simulink model "task8.1"  (R2023b)
settings: Solver=VariableStepAuto  StartTime=0.0  StopTime=2000  RelTol=1e-3
undefined symbols (not defined in the file or in its folder): SS_lat_lo8
libraries: slpidlib x5
settings Model: Creator=antonhendrickx  LastModifiedBy=antonhendrickx

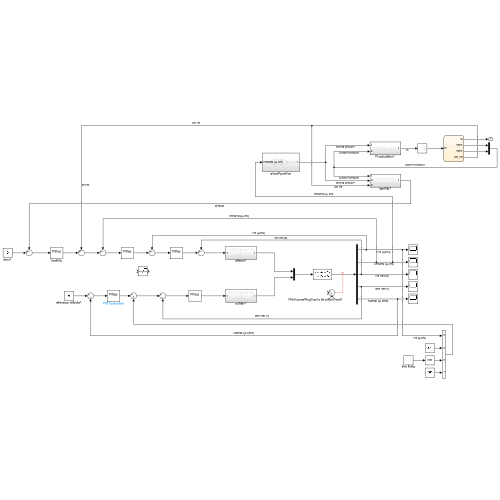
[thumbnail: Simulink's stored preview of the top-level diagram]
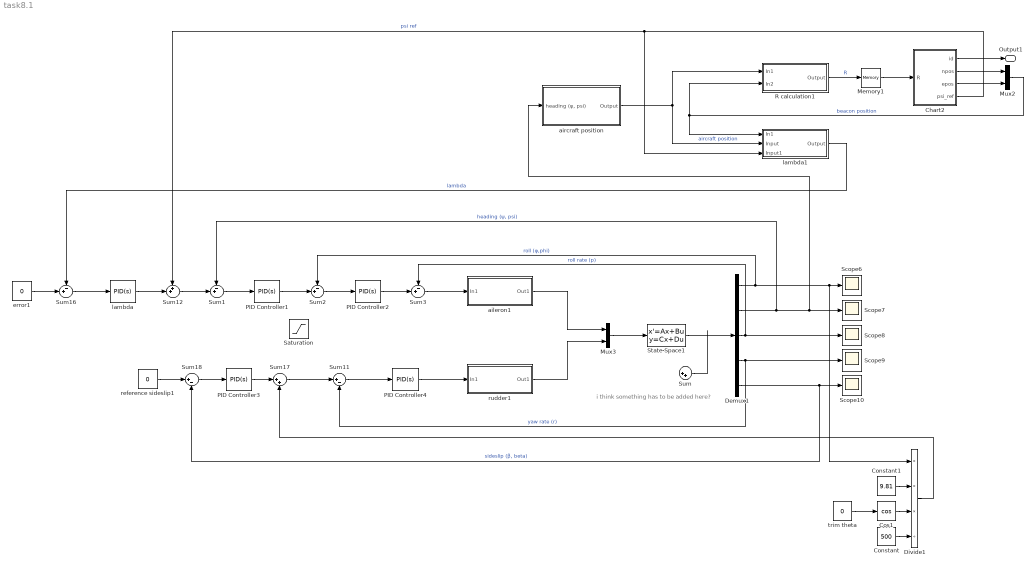
== system task8.1 ==
  note: i think something has to be added here?
  Chart2 : Stateflow chart  TreatAsAtomicUnit=on
  Constant : Constant  Value=500
  Constant1 : Constant  Value=9.81
  Cos1 : Trigonometry  Operator=cos
  Demux1 : Demux  Outputs=5
  Divide1 : Product  Inputs=***/
  Memory1 : Memory
  Mux2 : Mux  Inputs=2
  Mux3 : Mux  Inputs=2
  PID Controller{1..4} (4 alike) : slpidlib/PID Controller  Controller=PID  Form=Parallel  TimeDomain=Continuous-time  UseExternalTs=off  SampleTime=-1  IntegratorMethod=Forward Euler  FilterMethod=Forward Euler  ControllerParametersSource=internal  P=1  I=1  UseKiTs=off  D=0  N=100  UseFilter=on  TunerSelectOption=Transfer Function Based (PID Tuner App)  InitialConditionSource=internal  InitialConditionForIntegrator=0  InitialConditionForFilter=0  DifferentiatorICPrevScaledInput=0  ExternalReset=none  TrackingMode=off  Kt=1  LimitOutput=off  SatLimitsSource=internal  UpperSaturationLimit=inf  LowerSaturationLimit=-inf  LinearizeAsGain=on  AntiWindupMode=none  Kb=1  LimitIntegrator=off  UpperIntegratorSaturationLimit=inf  LowerIntegratorSaturationLimit=-inf  POutMin=[]  POutMax=[]  IOutMin=[]  IOutMax=[]  DOutMin=[]  DOutMax=[]  NOutMin=[]  NOutMax=[]  SumOutMin=[]  SumOutMax=[]  SaturationOutMin=[]  SaturationOutMax=[]  PParamMin=[]  PParamMax=[]  IParamMin=[]  IParamMax=[]  DParamMin=[]  DParamMax=[]  NParamMin=[]  NParamMax=[]  KbParamMin=[]  KbParamMax=[]  KtParamMin=[]  KtParamMax=[]  KbOutMin=[]  KbOutMax=[]  KtOutMin=[]  KtOutMax=[]  IntegratorOutMin=[]  IntegratorOutMax=[]  FilterOutMin=[]  FilterOutMax=[]  SumI1OutMin=[]  SumI1OutMax=[]  SumI2OutMin=[]  SumI2OutMax=[]  SumI3OutMin=[]  SumI3OutMax=[]  SumI4OutMin=[]  SumI4OutMax=[]  SumDOutMin=[]  SumDOutMax=[]  DifferentiatorOutMin=[]  DifferentiatorOutMax=[]  FilterDiffOutCoefMin=[]  FilterDiffOutCoefMax=[]  ReciprocalOutMin=[]  ReciprocalOutMax=[]  SumDenOutMin=[]  SumDenOutMax=[]  SumNumOutMin=[]  SumNumOutMax=[]  DivideOutMin=[]  DivideOutMax=[]  UdiffTsProdOutMin=[]  UdiffTsProdOutMax=[]  NTsProdOutMin=[]  NTsProdOutMax=[]  UintegralTsProdOutMin=[]  UintegralTsProdOutMax=[]  UngainTsProdOutMin=[]  UngainTsProdOutMax=[]  ClampingZeroOutDataTypeStr=Inherit: Inherit via back propagation  ClampingZeroOutMin=[]  ClampingZeroOutMax=[]  FilterDenConstantOutDataTypeStr=Inherit: Inherit via back propagation  FilterDenConstantOutMin=[]  FilterDenConstantOutMax=[]  PCopyOutDataTypeStr=Inherit: Inherit via back propagation  PCopyOutMin=[]  PCopyOutMax=[]  NCopyOutDataTypeStr=Inherit: Inherit via back propagation  NCopyOutMin=[]  NCopyOutMax=[]  IntegratorContinuousStateAttributes=''  IntegratorStateMustResolveToSignalObject=off  IntegratorRTWStateStorageClass=Auto  FilterContinuousStateAttributes=''  FilterStateMustResolveToSignalObject=off  FilterRTWStateStorageClass=Auto  ParallelPVariant=InternalParameters  IdealPVariant=Disabled  IVariant=InternalParameters  DVariant=InternalParameters  IntegratorVariant=Continuous  SatVariant=Disabled  AWVariant=Passthrough  PCopyVariant=Disabled  TRVariant=Disabled  FdbkBlocksVariant=Forward  IdealPFdbkVariant=Disabled  SatFdbkVariant=Disabled  DerivativeFilterVariant=ContFilter  NVariant=InternalParameters  NCopyVariant=Disabled  FilterICVariant=InternalICsFilter  IntegratorICVariant=InternalICs  ExternalResetVariant=Disabled  TRSumVariant=Passthrough  SumFdbkVariant=Disabled  SumVariant=Sum_PID  TsampFilterVariant=InternalTs  TsampNgainVariant=Passthrough  TsampIntegralVariant=Disabled_SignalSpec  ExternalSaturationOutDataTypeStr=Inherit: Same as second input
  R calculation1 : Subsystem
  Saturation : Saturate  UpperLimit=60  LowerLimit=-60
  Scope{6..10} (5 alike) : Scope
  State-Space1 : StateSpace  A=SS_lat_lo8.A  B=SS_lat_lo8.B  C=SS_lat_lo8.C  D=SS_lat_lo8.D  InitialCondition=0
  Sum : Sum  Inputs=|++
  Sum{1..3,16} (4 alike) : Sum  Inputs=-+|
  Sum11 : Sum  Inputs=|+-
  Sum12 : Sum  Inputs=++|
  Sum17 : Sum  Inputs=|++
  Sum18 : Sum  Inputs=|+-
  aileron1 : Subsystem
  aircraft position : Subsystem
  error1 : Constant  Value=0
  lambda : slpidlib/PID Controller  Controller=PID  Form=Parallel  TimeDomain=Continuous-time  UseExternalTs=off  SampleTime=-1  IntegratorMethod=Forward Euler  FilterMethod=Forward Euler  ControllerParametersSource=internal  P=1  I=1  UseKiTs=off  D=0  N=100  UseFilter=on  TunerSelectOption=Transfer Function Based (PID Tuner App)  InitialConditionSource=internal  InitialConditionForIntegrator=0  InitialConditionForFilter=0  DifferentiatorICPrevScaledInput=0  ExternalReset=none  TrackingMode=off  Kt=1  LimitOutput=off  SatLimitsSource=internal  UpperSaturationLimit=inf  LowerSaturationLimit=-inf  LinearizeAsGain=on  AntiWindupMode=none  Kb=1  LimitIntegrator=off  UpperIntegratorSaturationLimit=inf  LowerIntegratorSaturationLimit=-inf  POutMin=[]  POutMax=[]  IOutMin=[]  IOutMax=[]  DOutMin=[]  DOutMax=[]  NOutMin=[]  NOutMax=[]  SumOutMin=[]  SumOutMax=[]  SaturationOutMin=[]  SaturationOutMax=[]  PParamMin=[]  PParamMax=[]  IParamMin=[]  IParamMax=[]  DParamMin=[]  DParamMax=[]  NParamMin=[]  NParamMax=[]  KbParamMin=[]  KbParamMax=[]  KtParamMin=[]  KtParamMax=[]  KbOutMin=[]  KbOutMax=[]  KtOutMin=[]  KtOutMax=[]  IntegratorOutMin=[]  IntegratorOutMax=[]  FilterOutMin=[]  FilterOutMax=[]  SumI1OutMin=[]  SumI1OutMax=[]  SumI2OutMin=[]  SumI2OutMax=[]  SumI3OutMin=[]  SumI3OutMax=[]  SumI4OutMin=[]  SumI4OutMax=[]  SumDOutMin=[]  SumDOutMax=[]  DifferentiatorOutMin=[]  DifferentiatorOutMax=[]  FilterDiffOutCoefMin=[]  FilterDiffOutCoefMax=[]  ReciprocalOutMin=[]  ReciprocalOutMax=[]  SumDenOutMin=[]  SumDenOutMax=[]  SumNumOutMin=[]  SumNumOutMax=[]  DivideOutMin=[]  DivideOutMax=[]  UdiffTsProdOutMin=[]  UdiffTsProdOutMax=[]  NTsProdOutMin=[]  NTsProdOutMax=[]  UintegralTsProdOutMin=[]  UintegralTsProdOutMax=[]  UngainTsProdOutMin=[]  UngainTsProdOutMax=[]  ClampingZeroOutDataTypeStr=Inherit: Inherit via back propagation  ClampingZeroOutMin=[]  ClampingZeroOutMax=[]  FilterDenConstantOutDataTypeStr=Inherit: Inherit via back propagation  FilterDenConstantOutMin=[]  FilterDenConstantOutMax=[]  PCopyOutDataTypeStr=Inherit: Inherit via back propagation  PCopyOutMin=[]  PCopyOutMax=[]  NCopyOutDataTypeStr=Inherit: Inherit via back propagation  NCopyOutMin=[]  NCopyOutMax=[]  IntegratorContinuousStateAttributes=''  IntegratorStateMustResolveToSignalObject=off  IntegratorRTWStateStorageClass=Auto  FilterContinuousStateAttributes=''  FilterStateMustResolveToSignalObject=off  FilterRTWStateStorageClass=Auto  ParallelPVariant=InternalParameters  IdealPVariant=Disabled  IVariant=InternalParameters  DVariant=InternalParameters  IntegratorVariant=Continuous  SatVariant=Disabled  AWVariant=Passthrough  PCopyVariant=Disabled  TRVariant=Disabled  FdbkBlocksVariant=Forward  IdealPFdbkVariant=Disabled  SatFdbkVariant=Disabled  DerivativeFilterVariant=ContFilter  NVariant=InternalParameters  NCopyVariant=Disabled  FilterICVariant=InternalICsFilter  IntegratorICVariant=InternalICs  ExternalResetVariant=Disabled  TRSumVariant=Passthrough  SumFdbkVariant=Disabled  SumVariant=Sum_PID  TsampFilterVariant=InternalTs  TsampNgainVariant=Passthrough  TsampIntegralVariant=Disabled_SignalSpec  ExternalSaturationOutDataTypeStr=Inherit: Same as second input
  lambda1 : Subsystem
  reference sideslip1 : Constant  Value=0
  rudder1 : Subsystem
  trim theta : Constant  Value=0
  Output1 : Outport
  wires:
  Memory1/1 -> Chart2/1(R)
  Chart2/1(id) -> Output1/1
  Demux1/5 -> Scope10/1, Sum18/2  "sideslip (β, beta)"
  Chart2/3(epos) -> Mux2/2
  Demux1/2 -> Sum1/1, aircraft position/1("heading (ψ, psi)"), Scope7/1  "heading (ψ, psi)"
  Chart2/2(npos) -> Mux2/1
  State-Space1/1 -> Demux1/1
  Demux1/1 -> Sum2/1, Scope6/1, Divide1/1  "roll (φ,phi)"
  R calculation1/1(Output) -> Memory1/1  "R"
  Mux2/1 -> lambda1/1(In1), R calculation1/2(In2)  "beacon position"
  Demux1/3 -> Sum3/1, Scope8/1  "roll rate (p)"
  lambda1/1(Output) -> Sum16/1  "lambda"
  Chart2/4(psi_ref) -> lambda1/3(Input1), Sum12/1  "psi ref"
  Demux1/4 -> Scope9/1, Sum11/2  "yaw rate (r)"
  Sum16/1 -> lambda/1
  aileron1/1(Out1) -> Mux3/1
  error1/1 -> Sum16/2
  Sum12/1 -> Sum1/2
  Sum11/1 -> PID Controller4/1
  reference sideslip1/1 -> Sum18/1
  Sum18/1 -> PID Controller3/1
  Sum1/1 -> PID Controller1/1
  Sum17/1 -> Sum11/1
  Sum3/1 -> aileron1/1(In1)
  rudder1/1(Out1) -> Mux3/2
  Mux3/1 -> State-Space1/1
  Constant1/1 -> Divide1/2
  Cos1/1 -> Divide1/3
  Divide1/1 -> Sum17/2
  aircraft position/1(Output) -> lambda1/2(Input), R calculation1/1(In1)  "aircraft position"
  trim theta/1 -> Cos1/1
  Constant/1 -> Divide1/4
  lambda/1 -> Sum12/2
  PID Controller2/1 -> Sum3/2
  PID Controller3/1 -> Sum17/1
  PID Controller4/1 -> rudder1/1(In1)
  Sum/1 -> ?
  Sum2/1 -> PID Controller2/1
  PID Controller1/1 -> Sum2/2

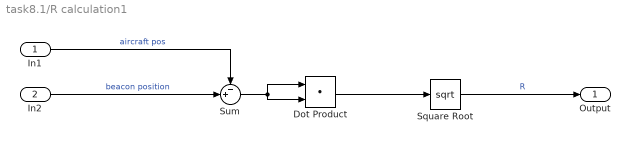
== system task8.1/R calculation1 ==
  In1 : Inport
  In2 : Inport  Port=2
  Dot Product : DotProduct  OutDataTypeStr=Inherit: Inherit via internal rule
  Square Root : Sqrt
  Sum : Sum  Inputs=-+|
  Output : Outport
  wires:
  In2/1 -> Sum/2  "beacon position"
  In1/1 -> Sum/1  "aircraft pos"
  Square Root/1 -> Output/1  "R"
  Dot Product/1 -> Square Root/1
  Sum/1 -> Dot Product/1, Dot Product/2

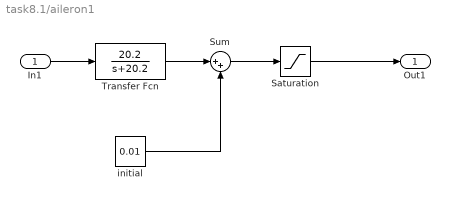
== system task8.1/aileron1 ==
  In1 : Inport
  Saturation : Saturate  UpperLimit=21.5  LowerLimit=-21.5
  Sum : Sum  Inputs=|++
  Transfer Fcn : TransferFcn  Numerator=[20.2]  Denominator=[1 20.2]
  initial : Constant  Value=0.01
  Out1 : Outport
  wires:
  Transfer Fcn/1 -> Sum/1
  Sum/1 -> Saturation/1
  Saturation/1 -> Out1/1
  In1/1 -> Transfer Fcn/1
  initial/1 -> Sum/2

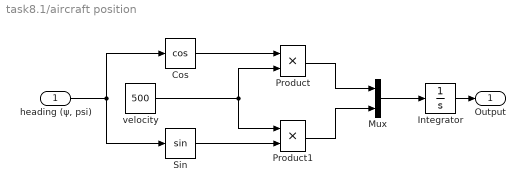
== system task8.1/aircraft position ==
  "heading (ψ, psi)" : Inport
  Cos : Trigonometry  Operator=cos
  Integrator : Integrator
  Mux : Mux  Inputs=2
  Product : Product
  Product1 : Product
  Sin : Trigonometry
  velocity : Constant  Value=500
  Output : Outport
  wires:
  Integrator/1 -> Output/1
  Sin/1 -> Product1/2
  Product1/1 -> Mux/2
  velocity/1 -> Product1/1, Product/2
  Product/1 -> Mux/1
  "heading (ψ, psi)"/1 -> Sin/1, Cos/1
  Cos/1 -> Product/1
  Mux/1 -> Integrator/1

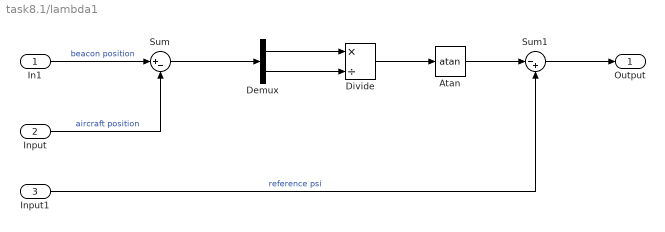
== system task8.1/lambda1 ==
  In1 : Inport
  Input : Inport  Port=2
  Input1 : Inport  Port=3
  Atan : Trigonometry  Operator=atan
  Demux : Demux  Outputs=2
  Divide : Product  Inputs=*/
  Sum : Sum  Inputs=|+-
  Sum1 : Sum  Inputs=|-+
  Output : Outport
  wires:
  In1/1 -> Sum/1  "beacon position"
  Demux/2 -> Divide/2
  Demux/1 -> Divide/1
  Divide/1 -> Atan/1
  Input/1 -> Sum/2  "aircraft position"
  Sum/1 -> Demux/1
  Input1/1 -> Sum1/2  "reference psi"
  Atan/1 -> Sum1/1
  Sum1/1 -> Output/1

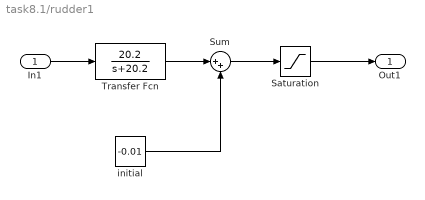
== system task8.1/rudder1 ==
  In1 : Inport
  Saturation : Saturate  UpperLimit=30  LowerLimit=-30
  Sum : Sum  Inputs=|++
  Transfer Fcn : TransferFcn  Numerator=[20.2]  Denominator=[1 20.2]
  initial : Constant  Value=-0.01
  Out1 : Outport
  wires:
  Transfer Fcn/1 -> Sum/1
  Sum/1 -> Saturation/1
  In1/1 -> Transfer Fcn/1
  initial/1 -> Sum/2
  Saturation/1 -> Out1/1

== stateflow chart task8.1/Chart2 ==
  settings: updateMethod=DISCRETE  sampleTime=0.1
  state beacon1
    id=1;
    npos=15000;
    epos=15000;
    psi_ref=45;
  state beacon2
    id=2;
    npos=0;
    epos=30000;
    psi_ref=135;
  state beacon3
    id=3;
    npos=-15000;
    epos=30000;
    psi_ref=180;
  state beacon4
    id=4;
    npos=-30000;
    epos=45000;
    psi_ref=135;
  state beacon5
    id=5;
    npos=0;
    epos=0;
    psi_ref=0;
  (default) -> beacon1
  beacon2 -> beacon3 : [R<5000]
  beacon3 -> beacon4 : [R<5000]
  beacon1 -> beacon2 : [R<5000]
  beacon4 -> beacon5 : [R<5000]
  beacon5 -> beacon1 : [R<5000]
  data: R input; id output; npos output; epos output; psi_ref output
